simulink model "fxpdemo_integrate"  (Simulink 7.6)
settings: Solver=ode5  SolverMode=SingleTasking  StartTime=0.0  StopTime=4  FixedStep=SampleTime/5  RelTol=1e-3  AbsTol=1e-6
PreLoadFcn:
  | preload_integrate
InitFcn:
  | ;
StartFcn:
  | ;
StopFcn:
  | ;
values from neighbouring files (symbols this model uses):
  SampleTime = 0.01    [preload_state_space.m]
undefined symbols (not defined in the file or in its folder): DiscIntNeverNeededParam
Description:
  | Fixed-Point Integrators
  | 
  | A comparison is provided between various fixed-point integrator realizations and an
  | equivalent floating point realization.
PreSaveFcn:
  | ;
CloseFcn:
  | close_integrate
settings Model: MinMaxOverflowLogging=MinMaxAndOverflow  Creator=The MathWorks Inc.  CovMetricSettings=d  ExtModeTrigMode=oneshot  ExtModeArmWhenConnect=off  ExtModeAutoUpdateStatusClock=off
settings DataIOCC: LimitDataPoints=off  TimeSaveName=timetest  OutputSaveName=youttest  SignalLoggingName=sigsOut
settings OptimizationCC: BooleanDataType=off  InlineInvariantSignals=on  InitFltsAndDblsToZero=on  EfficientMapNaN2IntZero=off
settings DebuggingCC: SaveWithParameterizedLinksMsg=none  SignalResolutionControl=TryResolveAllWithWarning  SolverPrmCheckMsg=none  MultiTaskDSMMsg=warning  MultiTaskCondExecSysMsg=none  SigSpecEnsureSampleTimeMsg=none  IntegerOverflowMsg=none  ParameterDowncastMsg=warning  ParameterOverflowMsg=warning  ParameterPrecisionLossMsg=none  StrictBusMsg=None
settings HardwareCC: TargetUnknown=on
settings RTWCC: IncludeERTFirstTime=on
settings GRTTargetCC: TargetFcnLib=ansi_tfl_tmw.mat

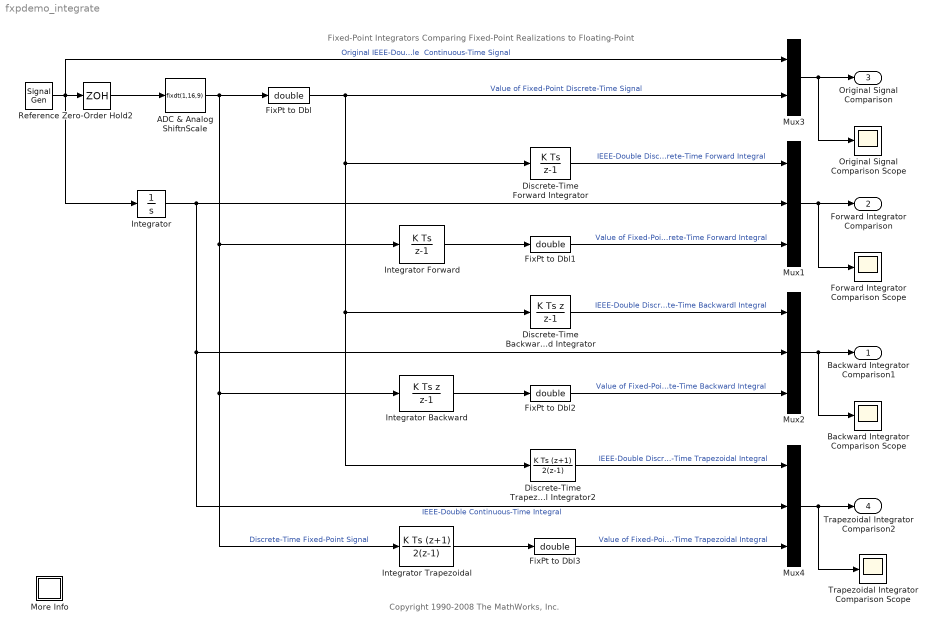
== system fxpdemo_integrate ==
  note: Copyright 1990-2008 The MathWorks, Inc.
  note: Fixed-Point Integrators
      | Comparing Fixed-Point Realizations to Floating-Point
  ADC & Analog ShiftnScale : DataTypeConversion  OutDataTypeStr=fixdt(1,16,9)  RndMeth=Nearest  SaturateOnIntegerOverflow=on  LockScale=on
  Backward Integrator Comparison Scope : Scope
      settings: TimeRange=4  YMin=-1.5  YMax=0.5  SaveName=ScopeData2
  Discrete-Time Backward Integrator : DiscreteIntegrator  IntegratorMethod=Integration: Backward Euler  SampleTime=SampleTime  ICPrevOutput=DiscIntNeverNeededParam  ICPrevScaledInput=DiscIntNeverNeededParam
  Discrete-Time Forward Integrator : DiscreteIntegrator  SampleTime=SampleTime  ICPrevOutput=DiscIntNeverNeededParam  ICPrevScaledInput=DiscIntNeverNeededParam
  Discrete-Time Trapezoidal Integrator2 : DiscreteIntegrator  IntegratorMethod=Integration: Trapezoidal  SampleTime=SampleTime  ICPrevOutput=DiscIntNeverNeededParam  ICPrevScaledInput=DiscIntNeverNeededParam
  FixPt to Dbl{,1..3} (4 alike) : DataTypeConversion  OutDataTypeStr=double
  Forward Integrator Comparison Scope : Scope
      settings: TimeRange=4  YMin=-1.5  YMax=0.5
  Integrator : Integrator
  Integrator Backward : DiscreteIntegrator  IntegratorMethod=Integration: Backward Euler  InitialCondition=0.0  InitialConditionMode=State only (most efficient)  SampleTime=-1  ICPrevOutput=DiscIntNeverNeededParam  ICPrevScaledInput=DiscIntNeverNeededParam
  Integrator Forward : DiscreteIntegrator  InitialCondition=0.0  InitialConditionMode=State only (most efficient)  SampleTime=-1  ICPrevOutput=DiscIntNeverNeededParam  ICPrevScaledInput=DiscIntNeverNeededParam
  Integrator Trapezoidal : DiscreteIntegrator  IntegratorMethod=Integration: Trapezoidal  InitialCondition=0.0 + 0.0  InitialConditionMode=State only (most efficient)  SampleTime=-1  ICPrevOutput=DiscIntNeverNeededParam  ICPrevScaledInput=DiscIntNeverNeededParam
  More Info : Subsystem
      settings: OpenFcn=showdemo(bdroot(gcs))
      mask Display: disp('?')
  Mux1 : Mux  Inputs=3
  Mux2 : Mux  Inputs=3
  Mux3 : Mux  Inputs=2
  Mux4 : Mux  Inputs=3
  Original Signal Comparison Scope : Scope
      settings: TimeRange=4  YMin=-1  YMax=1
  Reference : SignalGenerator  Amplitude=-1  Frequency=0.1*2.5
  Trapezoidal Integrator Comparison Scope : Scope
      settings: TimeRange=4  YMin=-1.5  YMax=0.5  SaveName=ScopeData3
  Zero-Order Hold2 : ZeroOrderHold  SampleTime=SampleTime
  Backward Integrator Comparison1 : Outport
  Forward Integrator Comparison : Outport  Port=2
  Original Signal Comparison : Outport  Port=3
  Trapezoidal Integrator Comparison2 : Outport  Port=4
  wires:
  Zero-Order Hold2/1 -> ADC & Analog ShiftnScale/1
  ADC & Analog ShiftnScale/1 -> FixPt to Dbl/1, Integrator Forward/1, Integrator Trapezoidal/1, Integrator Backward/1  "Discrete-Time Fixed-Point Signal"
  FixPt to Dbl/1 -> Mux3/2, Discrete-Time Trapezoidal Integrator2/1, Discrete-Time Backward Integrator/1, Discrete-Time Forward Integrator/1  "Value of Fixed-Point Discrete-Time Signal"
  Mux3/1 -> Original Signal Comparison/1, Original Signal Comparison Scope/1
  Reference/1 -> Mux3/1, Integrator/1, Zero-Order Hold2/1  "Original IEEE-Double  Continuous-Time Signal"
  FixPt to Dbl1/1 -> Mux1/3  "Value of Fixed-Point Discrete-Time Forward Integral"
  Mux1/1 -> Forward Integrator Comparison/1, Forward Integrator Comparison Scope/1
  Discrete-Time Forward Integrator/1 -> Mux1/1  "IEEE-Double Discrete-Time Forward Integral"
  Integrator Forward/1 -> FixPt to Dbl1/1
  Integrator/1 -> Mux1/2, Mux2/2, Mux4/2  "IEEE-Double Continuous-Time Integral"
  FixPt to Dbl2/1 -> Mux2/3  "Value of Fixed-Point Discrete-Time Backward Integral"
  Mux2/1 -> Backward Integrator Comparison1/1, Backward Integrator Comparison Scope/1
  Discrete-Time Backward Integrator/1 -> Mux2/1  "IEEE-Double Discrete-Time Backwardl Integral"
  Integrator Backward/1 -> FixPt to Dbl2/1
  FixPt to Dbl3/1 -> Mux4/3  "Value of Fixed-Point Discrete-Time Trapezoidal Integral"
  Mux4/1 -> Trapezoidal Integrator Comparison2/1, Trapezoidal Integrator Comparison Scope/1
  Discrete-Time Trapezoidal Integrator2/1 -> Mux4/1  "IEEE-Double Discrete-Time Trapezoidal Integral"
  Integrator Trapezoidal/1 -> FixPt to Dbl3/1

== system fxpdemo_integrate/More Info ==
